simulink model "tinygps_test"  (R2019a)
settings: Solver=FixedStepAuto  StartTime=0.0  StopTime=inf  FixedStep=0.01  RelTol=1e-3  EnableMultiTasking=on
settings Model: SimulationMode=external  ExtModeBatchMode=on  ExtModeEnableFloating=off  ExtModeTrigDuration=2  ExtModeTrigDurationFloating=20  Creator=Aliak  LastModifiedBy=Aliak
settings DataIOCC: ReturnWorkspaceOutputs=off
settings OptimizationCC: OptimizeBlockIOStorage=off  BufferReuse=off  GlobalBufferReuse=off  ExpressionFolding=off  EnableMemcpy=off  PassReuseOutputArgsAs=Individual arguments  LocalBlockOutputs=off  MaxStackSize=64  OptimizeDataStoreBuffers=off  BusAssignmentInplaceUpdate=off  OptimizationLevel=level0  OptimizationCustomize=off
settings DebuggingCC: ParameterTunabilityLossMsg=error  ArithmeticOperatorsInVariantConditions=warning
settings HardwareCC: ProdBitPerInt=16  ProdBitPerPointer=16  ProdBitPerSizeT=16  ProdBitPerPtrDiffT=16  ProdLargestAtomicFloat=None  ProdWordSize=8  ProdHWDeviceType=Atmel->AVR
settings SFSimCC: MATLABDynamicMemAlloc=off
settings RTWCC: SystemTargetFile=ert.tlc  HardwareBoard=Arduino Mega 2560  TLCOptions=-aInlineSetEventsForThisBaseRateFcn=TLC_FALSE -aSuppressMultiTaskScheduler=TLC_FALSE -aRateBasedStepFcn=1  TemplateMakefile=ert_default_tmf  GenerateReport=on  Toolchain=Arduino AVR  BuildConfiguration=Faster Runs  IncludeHyperlinkInReport=on  LaunchReport=on  CodeExecutionProfiling=on  CodeProfilingInstrumentation=detailed  GenerateTraceInfo=on  GenerateTraceReport=on  GenerateTraceReportSl=on  GenerateTraceReportSf=on  GenerateTraceReportEml=on
settings CodeAppCC: ForceParamTrailComments=on  IgnoreCustomStorageClasses=off  OperatorAnnotations=on  SimulinkDataObjDesc=on  SFDataObjDesc=on  InsertBlockDesc=on
settings ERTTargetCC: SupportAbsoluteTime=off  SupportNonFinite=off  SupportComplex=off

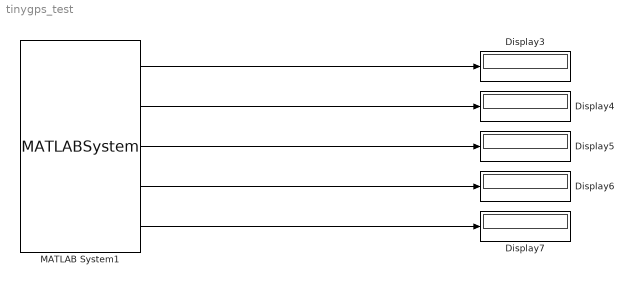
== system tinygps_test ==
  Display{3..7} (5 alike) : Display
  MATLAB System1 : MATLABSystem  System=TinyGPS  SimulateUsing=Code generation
      mask Type: TinyGPS
      mask Display:
      | disp('TinyGPS');
      | port_label('output',1,'lat');
      | port_label('output',2,'lon');
      | port_label('output',3,'speed');
      | port_label('output',4,'course');
      | port_label('output',5,'alt');
  wires:
  MATLAB System1/3 -> Display5/1
  MATLAB System1/5 -> Display7/1
  MATLAB System1/4 -> Display6/1
  MATLAB System1/2 -> Display4/1
  MATLAB System1/1 -> Display3/1
